simulink library "isi_correlator_lib"  (Simulink 7.0)
undefined symbols (not defined in the file): ROACH
libraries: xbsIndex_r4 x55, isi_correlator_lib x13, casper_library x8, xps_library x5
settings Model: Creator=wjm  LastModifiedBy=wjm

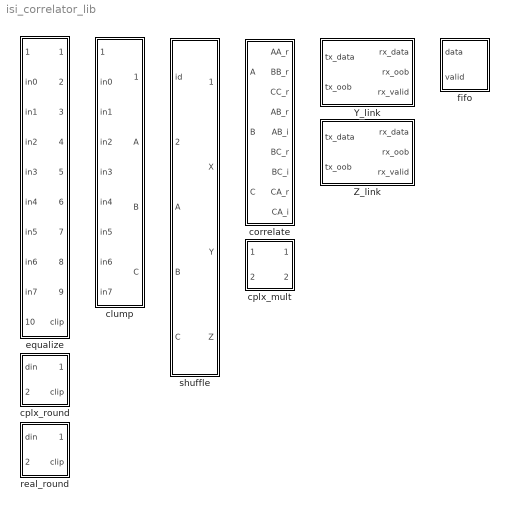
== system isi_correlator_lib ==
  Y_link : Subsystem
  Z_link : Subsystem
  clump : Subsystem
  correlate : Subsystem
  cplx_mult : Subsystem
  cplx_round : Subsystem
  equalize : Subsystem
  fifo : Subsystem
  real_round : Subsystem
  shuffle : Subsystem

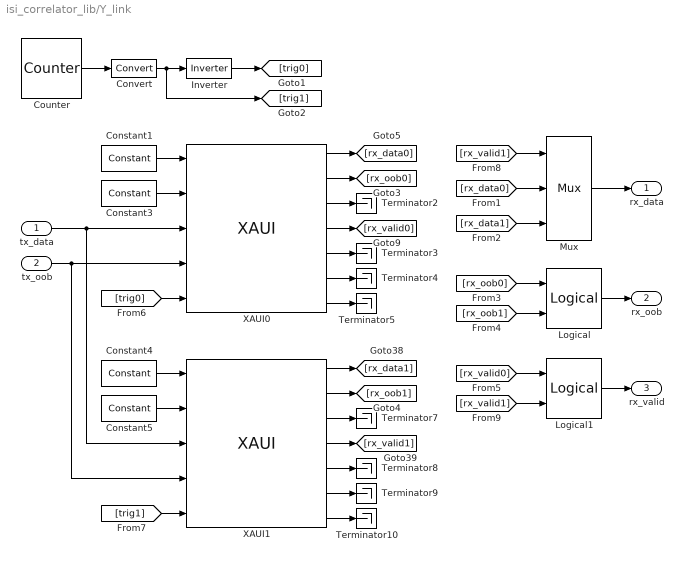
== system isi_correlator_lib/Y_link ==
  tx_data : Inport  OutDataType=sfix(16)  OutScaling=2^0
  tx_oob : Inport  Port=2  OutDataType=sfix(16)  OutScaling=2^0
  Constant1 : xbsIndex_r4/Constant  arith_type=Boolean  const=1  n_bits=1  bin_pt=0  explicit_period=on  period=1  equ=P=C  opselect=C  inp2=PCIN>>17  opr=+  inp1=P  carry=CIN  dbl_ovrd=off  block_type=constant
      settings: block_version=10.1.1
  Constant3 : xbsIndex_r4/Constant  arith_type=Boolean  const=0  n_bits=1  bin_pt=0  explicit_period=on  period=1  equ=P=C  opselect=C  inp2=PCIN>>17  opr=+  inp1=P  carry=CIN  dbl_ovrd=off  block_type=constant
      settings: block_version=10.1.1
  Constant4 : xbsIndex_r4/Constant  arith_type=Boolean  const=1  n_bits=1  bin_pt=0  explicit_period=on  period=1  equ=P=C  opselect=C  inp2=PCIN>>17  opr=+  inp1=P  carry=CIN  dbl_ovrd=off  block_type=constant
      settings: block_version=10.1.1
  Constant5 : xbsIndex_r4/Constant  arith_type=Boolean  const=0  n_bits=1  bin_pt=0  explicit_period=on  period=1  equ=P=C  opselect=C  inp2=PCIN>>17  opr=+  inp1=P  carry=CIN  dbl_ovrd=off  block_type=constant
      settings: block_version=10.1.1
  Convert : xbsIndex_r4/Convert  arith_type=Boolean  n_bits=16  bin_pt=14  quantization=Truncate  overflow=Wrap  latency=0  dbl_ovrd=off  pipeline=off  block_type=convert
      settings: block_version=10.1.3
  Counter : xbsIndex_r4/Counter  cnt_type=Free Running  cnt_to=Inf  operation=Up  start_count=0  cnt_by_val=1  arith_type=Unsigned  n_bits=1  bin_pt=0  load_pin=off  rst=off  en=off  explicit_period=on  period=1  dbl_ovrd=off  use_behavioral_HDL=off  use_rpm=off  implementation=Fabric  block_type=counter
  Inverter : xbsIndex_r4/Inverter  en=off  latency=0  dbl_ovrd=off  block_type=inv
  Logical : xbsIndex_r4/Logical  logical_function=OR  inputs=2  en=off  latency=0  precision=Full  arith_type=Unsigned  n_bits=16  bin_pt=0  align_bp=on  dbl_ovrd=off  block_type=logical
  Logical1 : xbsIndex_r4/Logical  logical_function=XOR  inputs=2  en=off  latency=0  precision=Full  arith_type=Unsigned  n_bits=16  bin_pt=0  align_bp=on  dbl_ovrd=off  block_type=logical
  Mux : xbsIndex_r4/Mux  inputs=2  en=off  latency=0  precision=Full  arith_type=Unsigned  n_bits=16  bin_pt=14  quantization=Truncate  overflow=Wrap  dbl_ovrd=off  block_type=mux
  Terminator{2..5,7..10} (8 alike) : Terminator
  XAUI0 : xps_library/XAUI  Tag=xps:xaui  SystemSampleTime=-1  demux=2  port=ROACH:0  show_param=off  pre_emph=3  swing=800
  XAUI1 : xps_library/XAUI  Tag=xps:xaui  SystemSampleTime=-1  demux=2  port=ROACH:1  show_param=off  pre_emph=3  swing=800
  rx_data : Outport  OutDataType=sfix(16)  OutScaling=2^0
  rx_oob : Outport  Port=2  OutDataType=sfix(16)  OutScaling=2^0
  rx_valid : Outport  Port=3  OutDataType=sfix(16)  OutScaling=2^0
  wires:
  [rx_valid0] -> Logical1/1
  [rx_valid1] -> Logical1/2
  Logical1/1 -> rx_valid/1
  [trig1] -> XAUI1/5
  [trig0] -> XAUI0/5
  Constant1/1 -> XAUI0/1
  Constant3/1 -> XAUI0/2
  Constant4/1 -> XAUI1/1
  Constant5/1 -> XAUI1/2
  XAUI0/2 -> [rx_oob0]
  XAUI0/3 -> Terminator2/1
  XAUI0/5 -> Terminator3/1
  XAUI0/6 -> Terminator4/1
  XAUI0/7 -> Terminator5/1
  XAUI1/7 -> Terminator10/1
  XAUI1/6 -> Terminator9/1
  XAUI1/5 -> Terminator8/1
  XAUI1/2 -> [rx_oob1]
  Counter/1 -> Convert/1
  Convert/1 -> Inverter/1, [trig1]
  Inverter/1 -> [trig0]
  tx_data/1 -> XAUI0/3, XAUI1/3
  tx_oob/1 -> XAUI0/4, XAUI1/4
  XAUI0/1 -> [rx_data0]
  XAUI0/4 -> [rx_valid0]
  XAUI1/1 -> [rx_data1]
  XAUI1/3 -> Terminator7/1
  XAUI1/4 -> [rx_valid1]
  [rx_oob0] -> Logical/1
  [rx_oob1] -> Logical/2
  Mux/1 -> rx_data/1
  Logical/1 -> rx_oob/1
  [rx_data0] -> Mux/2
  [rx_data1] -> Mux/3
  [rx_valid1] -> Mux/1

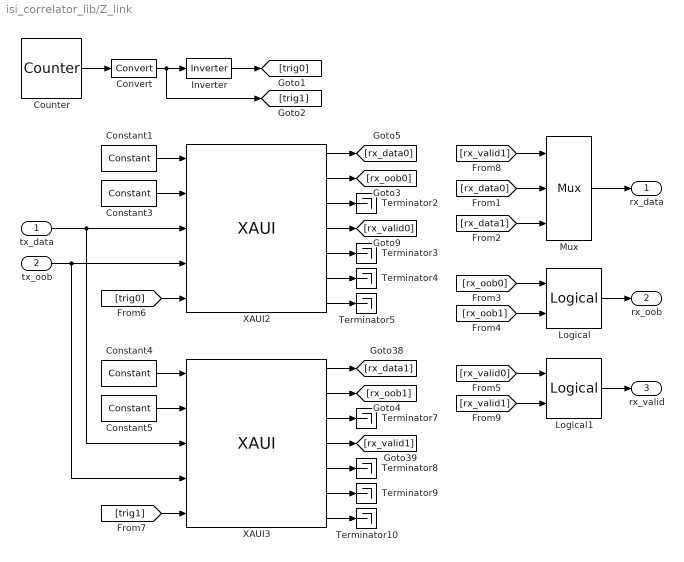
== system isi_correlator_lib/Z_link ==
  tx_data : Inport  OutDataType=sfix(16)  OutScaling=2^0
  tx_oob : Inport  Port=2  OutDataType=sfix(16)  OutScaling=2^0
  Constant1 : xbsIndex_r4/Constant  arith_type=Boolean  const=1  n_bits=1  bin_pt=0  explicit_period=on  period=1  equ=P=C  opselect=C  inp2=PCIN>>17  opr=+  inp1=P  carry=CIN  dbl_ovrd=off  block_type=constant
      settings: block_version=10.1.1
  Constant3 : xbsIndex_r4/Constant  arith_type=Boolean  const=0  n_bits=1  bin_pt=0  explicit_period=on  period=1  equ=P=C  opselect=C  inp2=PCIN>>17  opr=+  inp1=P  carry=CIN  dbl_ovrd=off  block_type=constant
      settings: block_version=10.1.1
  Constant4 : xbsIndex_r4/Constant  arith_type=Boolean  const=1  n_bits=1  bin_pt=0  explicit_period=on  period=1  equ=P=C  opselect=C  inp2=PCIN>>17  opr=+  inp1=P  carry=CIN  dbl_ovrd=off  block_type=constant
      settings: block_version=10.1.1
  Constant5 : xbsIndex_r4/Constant  arith_type=Boolean  const=0  n_bits=1  bin_pt=0  explicit_period=on  period=1  equ=P=C  opselect=C  inp2=PCIN>>17  opr=+  inp1=P  carry=CIN  dbl_ovrd=off  block_type=constant
      settings: block_version=10.1.1
  Convert : xbsIndex_r4/Convert  arith_type=Boolean  n_bits=16  bin_pt=14  quantization=Truncate  overflow=Wrap  latency=0  dbl_ovrd=off  pipeline=off  block_type=convert
      settings: block_version=10.1.3
  Counter : xbsIndex_r4/Counter  cnt_type=Free Running  cnt_to=Inf  operation=Up  start_count=0  cnt_by_val=1  arith_type=Unsigned  n_bits=1  bin_pt=0  load_pin=off  rst=off  en=off  explicit_period=on  period=1  dbl_ovrd=off  use_behavioral_HDL=off  use_rpm=off  implementation=Fabric  block_type=counter
  Inverter : xbsIndex_r4/Inverter  en=off  latency=0  dbl_ovrd=off  block_type=inv
  Logical : xbsIndex_r4/Logical  logical_function=OR  inputs=2  en=off  latency=0  precision=Full  arith_type=Unsigned  n_bits=16  bin_pt=0  align_bp=on  dbl_ovrd=off  block_type=logical
  Logical1 : xbsIndex_r4/Logical  logical_function=XOR  inputs=2  en=off  latency=0  precision=Full  arith_type=Unsigned  n_bits=16  bin_pt=0  align_bp=on  dbl_ovrd=off  block_type=logical
  Mux : xbsIndex_r4/Mux  inputs=2  en=off  latency=0  precision=Full  arith_type=Unsigned  n_bits=16  bin_pt=14  quantization=Truncate  overflow=Wrap  dbl_ovrd=off  block_type=mux
  Terminator{2..5,7..10} (8 alike) : Terminator
  XAUI2 : xps_library/XAUI  Tag=xps:xaui  SystemSampleTime=-1  demux=2  port=ROACH:2  show_param=off  pre_emph=3  swing=800
  XAUI3 : xps_library/XAUI  Tag=xps:xaui  SystemSampleTime=-1  demux=2  port=ROACH:3  show_param=off  pre_emph=3  swing=800
  rx_data : Outport  OutDataType=sfix(16)  OutScaling=2^0
  rx_oob : Outport  Port=2  OutDataType=sfix(16)  OutScaling=2^0
  rx_valid : Outport  Port=3  OutDataType=sfix(16)  OutScaling=2^0
  wires:
  [rx_valid0] -> Logical1/1
  [rx_valid1] -> Logical1/2
  Logical1/1 -> rx_valid/1
  [trig1] -> XAUI3/5
  [trig0] -> XAUI2/5
  Constant1/1 -> XAUI2/1
  Constant3/1 -> XAUI2/2
  Constant4/1 -> XAUI3/1
  Constant5/1 -> XAUI3/2
  XAUI2/2 -> [rx_oob0]
  XAUI2/3 -> Terminator2/1
  XAUI2/5 -> Terminator3/1
  XAUI2/6 -> Terminator4/1
  XAUI2/7 -> Terminator5/1
  XAUI3/7 -> Terminator10/1
  XAUI3/6 -> Terminator9/1
  XAUI3/5 -> Terminator8/1
  XAUI3/2 -> [rx_oob1]
  Counter/1 -> Convert/1
  Convert/1 -> Inverter/1, [trig1]
  Inverter/1 -> [trig0]
  tx_data/1 -> XAUI2/3, XAUI3/3
  tx_oob/1 -> XAUI2/4, XAUI3/4
  XAUI2/1 -> [rx_data0]
  XAUI2/4 -> [rx_valid0]
  XAUI3/1 -> [rx_data1]
  XAUI3/3 -> Terminator7/1
  XAUI3/4 -> [rx_valid1]
  [rx_oob0] -> Logical/1
  [rx_oob1] -> Logical/2
  Mux/1 -> rx_data/1
  Logical/1 -> rx_oob/1
  [rx_data0] -> Mux/2
  [rx_data1] -> Mux/3
  [rx_valid1] -> Mux/1

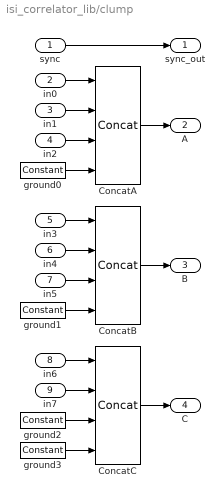
== system isi_correlator_lib/clump ==
  sync : Inport
  in0 : Inport  Port=2
  in1 : Inport  Port=3
  in2 : Inport  Port=4
  in3 : Inport  Port=5
  in4 : Inport  Port=6
  in5 : Inport  Port=7
  in6 : Inport  Port=8
  in7 : Inport  Port=9
  ConcatA : xbsIndex_r4/Concat  num_inputs=4  dbl_ovrd=off  block_type=concat
      settings: block_version=10.1.1
  ConcatB : xbsIndex_r4/Concat  num_inputs=4  dbl_ovrd=off  block_type=concat
      settings: block_version=10.1.1
  ConcatC : xbsIndex_r4/Concat  num_inputs=4  dbl_ovrd=off  block_type=concat
      settings: block_version=10.1.1
  ground{0..3} (4 alike) : xbsIndex_r4/Constant  arith_type=Unsigned  const=0  n_bits=8  bin_pt=0  explicit_period=on  period=1  equ=P=C  opselect=C  inp2=PCIN>>17  opr=+  inp1=P  carry=CIN  dbl_ovrd=off  block_type=constant
      settings: block_version=10.1.1
  sync_out : Outport
  A : Outport  Port=2
  B : Outport  Port=3
  C : Outport  Port=4
  wires:
  ConcatC/1 -> C/1
  ConcatB/1 -> B/1
  ConcatA/1 -> A/1
  ground3/1 -> ConcatC/4
  ground2/1 -> ConcatC/3
  in7/1 -> ConcatC/2
  in6/1 -> ConcatC/1
  ground1/1 -> ConcatB/4
  in5/1 -> ConcatB/3
  in4/1 -> ConcatB/2
  in3/1 -> ConcatB/1
  ground0/1 -> ConcatA/4
  in2/1 -> ConcatA/3
  in1/1 -> ConcatA/2
  in0/1 -> ConcatA/1
  sync/1 -> sync_out/1

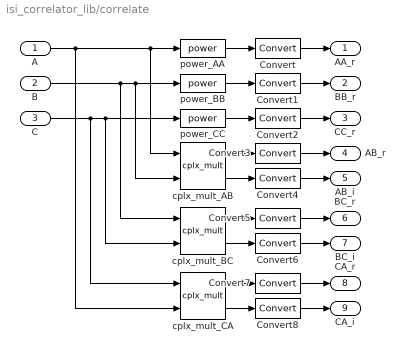
== system isi_correlator_lib/correlate ==
  A : Inport  OutDataType=sfix(16)  OutScaling=2^0
  B : Inport  Port=2  OutDataType=sfix(16)  OutScaling=2^0
  C : Inport  Port=3  OutDataType=sfix(16)  OutScaling=2^0
  Convert{,1..8} (9 alike) : xbsIndex_r4/Convert  arith_type="Signed  (2's comp)"  n_bits=8  bin_pt=7  quantization=Truncate  overflow=Wrap  latency=0  dbl_ovrd=off  pipeline=off  block_type=convert
      settings: block_version=10.1.3
  cplx_mult_AB : isi_correlator_lib/cplx_mult  SystemSampleTime=-1
  cplx_mult_BC : isi_correlator_lib/cplx_mult  SystemSampleTime=-1
  cplx_mult_CA : isi_correlator_lib/cplx_mult  SystemSampleTime=-1
  power_AA : casper_library/Misc/power  SystemSampleTime=-1  BitWidth=8
  power_BB : casper_library/Misc/power  SystemSampleTime=-1  BitWidth=8
  power_CC : casper_library/Misc/power  SystemSampleTime=-1  BitWidth=8
  AA_r : Outport  OutDataType=sfix(16)  OutScaling=2^0
  BB_r : Outport  Port=2  OutDataType=sfix(16)  OutScaling=2^0
  CC_r : Outport  Port=3  OutDataType=sfix(16)  OutScaling=2^0
  AB_r : Outport  Port=4  OutDataType=sfix(16)  OutScaling=2^0
  AB_i : Outport  Port=5  OutDataType=sfix(16)  OutScaling=2^0
  BC_r : Outport  Port=6  OutDataType=sfix(16)  OutScaling=2^0
  BC_i : Outport  Port=7  OutDataType=sfix(16)  OutScaling=2^0
  CA_r : Outport  Port=8  OutDataType=sfix(16)  OutScaling=2^0
  CA_i : Outport  Port=9  OutDataType=sfix(16)  OutScaling=2^0
  wires:
  Convert8/1 -> CA_i/1
  Convert7/1 -> CA_r/1
  Convert6/1 -> BC_i/1
  Convert5/1 -> BC_r/1
  Convert4/1 -> AB_i/1
  Convert3/1 -> AB_r/1
  Convert2/1 -> CC_r/1
  Convert1/1 -> BB_r/1
  Convert/1 -> AA_r/1
  cplx_mult_CA/2 -> Convert8/1
  cplx_mult_CA/1 -> Convert7/1
  cplx_mult_BC/2 -> Convert6/1
  cplx_mult_BC/1 -> Convert5/1
  cplx_mult_AB/2 -> Convert4/1
  cplx_mult_AB/1 -> Convert3/1
  power_CC/1 -> Convert2/1
  power_BB/1 -> Convert1/1
  power_AA/1 -> Convert/1
  A/1 -> cplx_mult_AB/1, power_AA/1, cplx_mult_CA/2
  B/1 -> cplx_mult_AB/2, power_BB/1, cplx_mult_BC/1
  C/1 -> cplx_mult_BC/2, power_CC/1, cplx_mult_CA/1

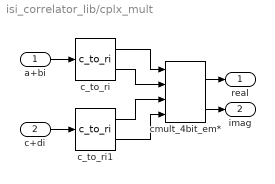
== system isi_correlator_lib/cplx_mult ==
  a+bi : Inport  OutDataType=sfix(16)  OutScaling=2^0
  c+di : Inport  Port=2  OutDataType=sfix(16)  OutScaling=2^0
  c_to_ri : casper_library/Misc/c_to_ri  SystemSampleTime=-1  n_bits=8  bin_pt=7
      settings: AttributesFormatString=8_7 r/i
  c_to_ri1 : casper_library/Misc/c_to_ri  SystemSampleTime=-1  n_bits=8  bin_pt=7
      settings: AttributesFormatString=8_7 r/i
  cmult_4bit_em* : casper_library/Multipliers/cmult_4bit_em*  SystemSampleTime=-1  mult_latency=3  add_latency=2
  real : Outport  OutDataType=sfix(16)  OutScaling=2^0
  imag : Outport  Port=2  OutDataType=sfix(16)  OutScaling=2^0
  wires:
  cmult_4bit_em*/2 -> imag/1
  cmult_4bit_em*/1 -> real/1
  a+bi/1 -> c_to_ri/1
  c_to_ri/1 -> cmult_4bit_em*/1
  c+di/1 -> c_to_ri1/1
  c_to_ri1/2 -> cmult_4bit_em*/4
  c_to_ri/2 -> cmult_4bit_em*/2
  c_to_ri1/1 -> cmult_4bit_em*/3

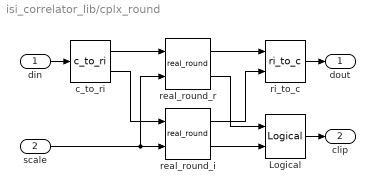
== system isi_correlator_lib/cplx_round ==
  din : Inport  OutDataType=sfix(16)  OutScaling=2^0
  scale : Inport  Port=2  OutDataType=sfix(16)  OutScaling=2^0
  Logical : xbsIndex_r4/Logical  logical_function=OR  inputs=2  en=off  latency=2  precision=Full  arith_type=Unsigned  n_bits=8  bin_pt=2  align_bp=on  dbl_ovrd=off  block_type=logical
      settings: xl_area=[0, 0, 0, 0, 0, 0, 0]
  c_to_ri : casper_library/Misc/c_to_ri  SystemSampleTime=-1  n_bits=8  bin_pt=7
      settings: AttributesFormatString=8_7 r/i
  real_round_i : isi_correlator_lib/real_round  SystemSampleTime=-1
  real_round_r : isi_correlator_lib/real_round  SystemSampleTime=-1
  ri_to_c : casper_library/Misc/ri_to_c  SystemSampleTime=-1
  dout : Outport  OutDataType=sfix(16)  OutScaling=2^0
  clip : Outport  Port=2  OutDataType=sfix(16)  OutScaling=2^0
  wires:
  c_to_ri/2 -> real_round_i/1
  c_to_ri/1 -> real_round_r/1
  din/1 -> c_to_ri/1
  real_round_i/1 -> ri_to_c/2
  real_round_r/1 -> ri_to_c/1
  scale/1 -> real_round_i/2, real_round_r/2
  real_round_i/2 -> Logical/2
  real_round_r/2 -> Logical/1
  ri_to_c/1 -> dout/1
  Logical/1 -> clip/1

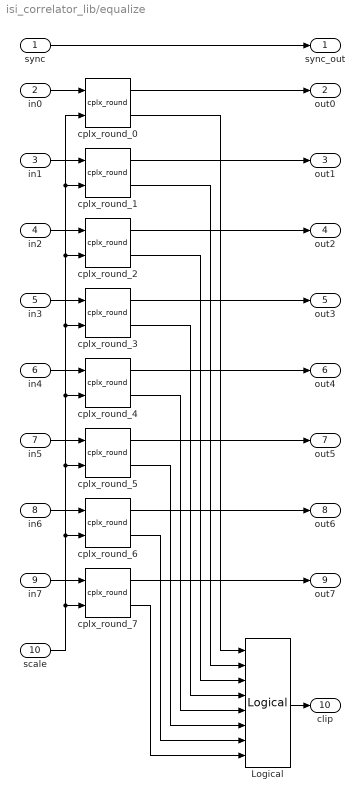
== system isi_correlator_lib/equalize ==
  sync : Inport
  in0 : Inport  Port=2
  in1 : Inport  Port=3
  in2 : Inport  Port=4
  in3 : Inport  Port=5
  in4 : Inport  Port=6
  in5 : Inport  Port=7
  in6 : Inport  Port=8
  in7 : Inport  Port=9
  scale : Inport  Port=10
  Logical : xbsIndex_r4/Logical  logical_function=OR  inputs=8  en=off  latency=0  precision=Full  arith_type=Unsigned  n_bits=16  bin_pt=0  align_bp=on  dbl_ovrd=off  block_type=logical
  cplx_round_{0..7} (8 alike) : isi_correlator_lib/cplx_round  SystemSampleTime=-1
  sync_out : Outport
  out0 : Outport  Port=2
  out1 : Outport  Port=3
  out2 : Outport  Port=4
  out3 : Outport  Port=5
  out4 : Outport  Port=6
  out5 : Outport  Port=7
  out6 : Outport  Port=8
  out7 : Outport  Port=9
  clip : Outport  Port=10
  wires:
  sync/1 -> sync_out/1
  scale/1 -> cplx_round_0/2, cplx_round_1/2, cplx_round_2/2, cplx_round_3/2, cplx_round_4/2, cplx_round_5/2, cplx_round_6/2, cplx_round_7/2
  in0/1 -> cplx_round_0/1
  in1/1 -> cplx_round_1/1
  in2/1 -> cplx_round_2/1
  in3/1 -> cplx_round_3/1
  in4/1 -> cplx_round_4/1
  in5/1 -> cplx_round_5/1
  in6/1 -> cplx_round_6/1
  in7/1 -> cplx_round_7/1
  cplx_round_0/1 -> out0/1
  cplx_round_1/1 -> out1/1
  cplx_round_2/1 -> out2/1
  cplx_round_3/1 -> out3/1
  cplx_round_4/1 -> out4/1
  cplx_round_5/1 -> out5/1
  cplx_round_6/1 -> out6/1
  cplx_round_7/1 -> out7/1
  cplx_round_7/2 -> Logical/8
  cplx_round_6/2 -> Logical/7
  cplx_round_5/2 -> Logical/6
  cplx_round_4/2 -> Logical/5
  cplx_round_3/2 -> Logical/4
  cplx_round_2/2 -> Logical/3
  cplx_round_1/2 -> Logical/2
  cplx_round_0/2 -> Logical/1
  Logical/1 -> clip/1

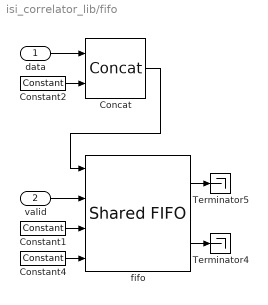
== system isi_correlator_lib/fifo ==
  data : Inport
  valid : Inport  Port=2
  Concat : xbsIndex_r4/Concat  num_inputs=2  dbl_ovrd=off  block_type=concat
      settings: block_version=10.1.3
  Constant1 : xbsIndex_r4/Constant  arith_type=Boolean  const=0  n_bits=1  bin_pt=0  explicit_period=on  period=1  equ=P=C  opselect=C  inp2=PCIN>>17  opr=+  inp1=P  carry=CIN  dbl_ovrd=off  block_type=constant
      settings: block_version=10.1.1
  Constant2 : xbsIndex_r4/Constant  arith_type=Unsigned  const=0  n_bits=4  bin_pt=0  explicit_period=on  period=1  equ=P=C  opselect=C  inp2=PCIN>>17  opr=+  inp1=P  carry=CIN  dbl_ovrd=off  block_type=constant
      settings: block_version=10.1.1
  Constant4 : xbsIndex_r4/Constant  arith_type=Boolean  const=0  n_bits=1  bin_pt=0  explicit_period=on  period=1  equ=P=C  opselect=C  inp2=PCIN>>17  opr=+  inp1=P  carry=CIN  dbl_ovrd=off  block_type=constant
      settings: block_version=10.1.1
  Terminator4 : Terminator
  Terminator5 : Terminator
  fifo : xps_library/Shared FIFO  Tag=xps:fifo  SystemSampleTime=-1  io_dir=To Processor  arith_type=Unsigned  data_width=256  data_bin_pt=0  fifo_length=512
  wires:
  fifo/1 -> Terminator5/1
  fifo/2 -> Terminator4/1
  Constant1/1 -> fifo/3
  Constant4/1 -> fifo/4
  data/1 -> Concat/1
  Constant2/1 -> Concat/2
  valid/1 -> fifo/2
  Concat/1 -> fifo/1

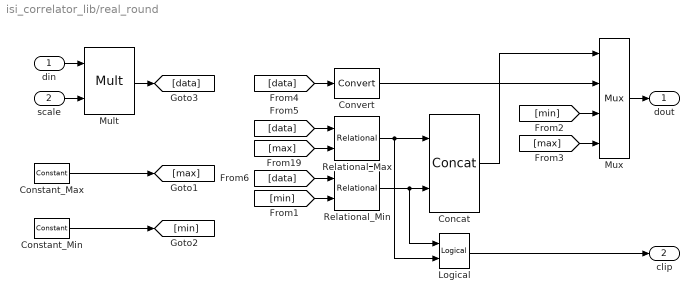
== system isi_correlator_lib/real_round ==
  din : Inport  OutDataType=sfix(16)  OutScaling=2^0
  scale : Inport  Port=2  OutDataType=sfix(16)  OutScaling=2^0
  Concat : xbsIndex_r4/Concat  num_inputs=2  dbl_ovrd=off  block_type=concat
      settings: block_version=10.1.3
  Constant_Max : xbsIndex_r4/Constant  arith_type=Signed (2's comp)  const=7/8  n_bits=4  bin_pt=3  explicit_period=on  period=1  equ=P=C  opselect=C  inp2=PCIN>>17  opr=+  inp1=P  carry=CIN  dbl_ovrd=off  block_type=constant
  Constant_Min : xbsIndex_r4/Constant  arith_type=Signed (2's comp)  const=-7/8  n_bits=4  bin_pt=3  explicit_period=on  period=1  equ=P=C  opselect=C  inp2=PCIN>>17  opr=+  inp1=P  carry=CIN  dbl_ovrd=off  block_type=constant
  Convert : xbsIndex_r4/Convert  arith_type="Signed  (2's comp)"  n_bits=4  bin_pt=3  quantization="Round  (unbiased: Even Values)"  overflow=Wrap  latency=2  dbl_ovrd=off  pipeline=off  block_type=convert
      settings: xl_area=[0, 0, 0, 0, 0, 0, 0]  block_version=10.1.3
  Logical : xbsIndex_r4/Logical  logical_function=OR  inputs=2  en=off  latency=2  precision=Full  arith_type=Unsigned  n_bits=8  bin_pt=2  align_bp=on  dbl_ovrd=off  block_type=logical
      settings: xl_area=[0, 0, 0, 0, 0, 0, 0]
  Mult : xbsIndex_r4/Mult  precision=Full  arith_type="Signed  (2's comp)"  n_bits=16  bin_pt=14  quantization=Truncate  overflow=Wrap  en=off  latency=2  dbl_ovrd=off  use_behavioral_HDL=off  use_embedded=on  opt=Speed  optimum_pipeline=off  pipeline=on  use_rpm=on  placement_style=Triangular  block_type=mult
      settings: infoedit=Hardware notes: To use the internal pipeline stage of the dedicated multiplier you must select 'Pipeline for maximum performance'.  block_version=10.1.3
  Mux : xbsIndex_r4/Mux  inputs=3  en=off  latency=0  precision=Full  arith_type="Signed  (2's comp)"  n_bits=8  bin_pt=2  quantization=Truncate  overflow=Wrap  dbl_ovrd=off  block_type=mux
      settings: xl_area=[0, 0, 0, 0, 0, 0, 0]
  Relational_Max : xbsIndex_r4/Relational  mode=a>b  en=off  latency=2  dbl_ovrd=off  block_type=relational
      settings: xl_area=[0, 0, 0, 0, 0, 0, 0]  block_version=10.1.3
  Relational_Min : xbsIndex_r4/Relational  mode=a<b  en=off  latency=2  dbl_ovrd=off  block_type=relational
      settings: xl_area=[0, 0, 0, 0, 0, 0, 0]  block_version=10.1.3
  dout : Outport  OutDataType=sfix(16)  OutScaling=2^0
  clip : Outport  Port=2  OutDataType=sfix(16)  OutScaling=2^0
  wires:
  Convert/1 -> Mux/2
  din/1 -> Mult/1
  scale/1 -> Mult/2
  Constant_Max/1 -> [max]
  Constant_Min/1 -> [min]
  Relational_Max/1 -> Concat/1, Logical/2
  Relational_Min/1 -> Concat/2, Logical/1
  Concat/1 -> Mux/1
  [min] -> Mux/3
  [max] -> Mux/4
  Mux/1 -> dout/1
  Logical/1 -> clip/1
  [min] -> Relational_Min/2
  [data] -> Relational_Min/1
  [max] -> Relational_Max/2
  [data] -> Relational_Max/1
  Mult/1 -> [data]
  [data] -> Convert/1

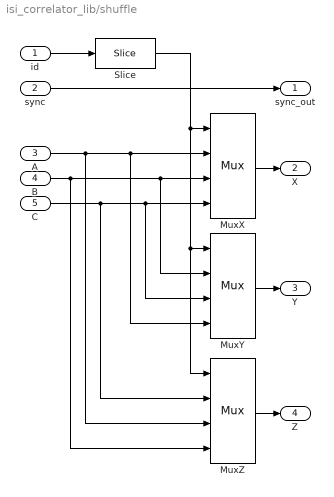
== system isi_correlator_lib/shuffle ==
  id : Inport  OutDataType=sfix(16)  OutScaling=2^0
  sync : Inport  Port=2  OutDataType=sfix(16)  OutScaling=2^0
  A : Inport  Port=3  OutDataType=sfix(16)  OutScaling=2^0
  B : Inport  Port=4  OutDataType=sfix(16)  OutScaling=2^0
  C : Inport  Port=5  OutDataType=sfix(16)  OutScaling=2^0
  MuxX : xbsIndex_r4/Mux  inputs=3  en=off  latency=0  precision=Full  arith_type=Unsigned  n_bits=16  bin_pt=14  quantization=Truncate  overflow=Wrap  dbl_ovrd=off  block_type=mux
  MuxY : xbsIndex_r4/Mux  inputs=3  en=off  latency=0  precision=Full  arith_type=Unsigned  n_bits=16  bin_pt=14  quantization=Truncate  overflow=Wrap  dbl_ovrd=off  block_type=mux
  MuxZ : xbsIndex_r4/Mux  inputs=3  en=off  latency=0  precision=Full  arith_type=Unsigned  n_bits=16  bin_pt=14  quantization=Truncate  overflow=Wrap  dbl_ovrd=off  block_type=mux
  Slice : xbsIndex_r4/Slice  nbits=2  boolean_output=off  mode=Lower Bit Location + Width  bit1=0  base1=MSB of Input  bit0=2  base0=LSB of Input  dbl_ovrd=off  block_type=slice
      settings: infoedit="Extracts a given range of bits from each input sample and presents it at the output.  The output type is ordinarily unsigned with binary point at zero, but can be Boolean when the slice is one bit wide.<P><P>Hardware notes: In hardware this block costs nothing."  block_version=10.1.3
  sync_out : Outport  OutDataType=sfix(16)  OutScaling=2^0
  X : Outport  Port=2  OutDataType=sfix(16)  OutScaling=2^0
  Y : Outport  Port=3  OutDataType=sfix(16)  OutScaling=2^0
  Z : Outport  Port=4  OutDataType=sfix(16)  OutScaling=2^0
  wires:
  MuxX/1 -> X/1
  MuxY/1 -> Y/1
  MuxZ/1 -> Z/1
  id/1 -> Slice/1
  A/1 -> MuxX/2, MuxY/4, MuxZ/3
  B/1 -> MuxX/3, MuxY/2, MuxZ/4
  C/1 -> MuxX/4, MuxY/3, MuxZ/2
  Slice/1 -> MuxZ/1, MuxY/1, MuxX/1
  sync/1 -> sync_out/1
